simulink model "estuarymodel"  (R2021a)
settings: Solver=VariableStepAuto  StartTime=0.0  StopTime=100  RelTol=1e-3
values from neighbouring files (symbols this model uses):
  initial_river_volume = 200    [estuarymodel.mat]
  initial_sea_volume = 200    [estuarymodel.mat]
  r_evap = 5    [estuarymodel.mat]
  rho_river = 1000    [estuarymodel.mat]
  rho_sea = 1025    [estuarymodel.mat]
  RiverFlow = 10    [estuarymodel.mat]
  SeaFlow = 10    [estuarymodel.mat]
settings Model: Creator=dylan  LastModifiedBy=dylan

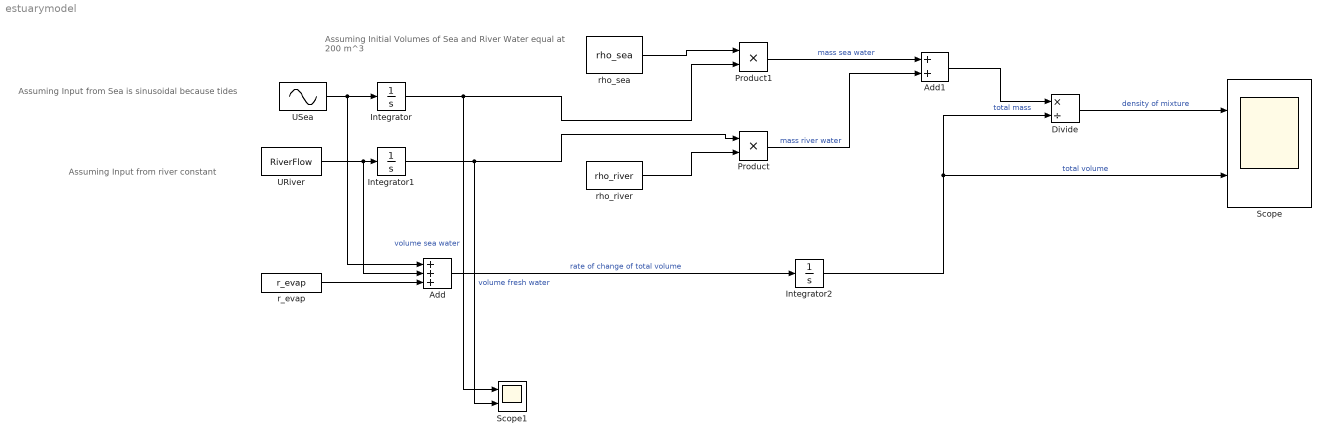
== system estuarymodel ==
  note: Assuming Initial Volumes of Sea and River Water equal
      | at 200 m^3
  note: Assuming Input from river constant
  note: Assuming Input from Sea is sinusoidal because tides
  Add : Sum  Inputs=+++
  Add1 : Sum
  Divide : Product  Inputs=*/
  Integrator : Integrator  InitialCondition=initial_sea_volume
  Integrator1 : Integrator  InitialCondition=initial_river_volume
  Integrator2 : Integrator
  Product : Product
  Product1 : Product
  Scope : Scope  NumInputPorts=2
  Scope1 : Scope  NumInputPorts=2
  URiver : Constant  Value=RiverFlow
  USea : Sin  Amplitude=SeaFlow  Frequency=1/12  SampleTime=0
  r_evap : Constant  Value=r_evap
  rho_river : Constant  Value=rho_river
  rho_sea : Constant  Value=rho_sea
  wires:
  URiver/1 -> Add/2, Integrator1/1
  Integrator/1 -> Product1/2, Scope1/1  "volume sea water"
  Integrator1/1 -> Scope1/2, Product/1  "volume fresh water"
  Add/1 -> Integrator2/1  "rate of change of total volume"
  r_evap/1 -> Add/3
  rho_river/1 -> Product/2
  rho_sea/1 -> Product1/1
  Product/1 -> Add1/2  "mass river water"
  Product1/1 -> Add1/1  "mass sea water"
  Integrator2/1 -> Divide/2, Scope/2  "total volume"
  Add1/1 -> Divide/1  "total mass"
  Divide/1 -> Scope/1  "density of mixture"
  USea/1 -> Add/1, Integrator/1
